simulink model "DebuggingModel_1"  (R2022b)
settings: Solver=VariableStepAuto  StartTime=0.0  StopTime=10.0  RelTol=1e-3
model workspace (MAT data in the model file):
  accumulated_data = Simulink.Signal
  accumulated_data.DataType = 'auto'
  accumulated_data.Dimensions = -1
  accumulated_data.DimensionsMode = 'auto'
  accumulated_data.Complexity = 'auto'
  accumulated_data.SampleTime = -1
  accumulated_data.SamplingMode = 'auto'
  lambda_cost = Simulink.Signal
  lambda_cost.DataType = 'double'
  lambda_cost.Dimensions = -1
  lambda_cost.DimensionsMode = 'auto'
  lambda_cost.Complexity = 'auto'
  lambda_cost.SampleTime = -1
  lambda_cost.SamplingMode = 'auto'
  lambda_cost.InitialValue = '0'
  total_cost = Simulink.Signal
  total_cost.DataType = 'auto'
  total_cost.Dimensions = -1
  total_cost.DimensionsMode = 'auto'
  total_cost.Complexity = 'auto'
  total_cost.SampleTime = -1
  total_cost.SamplingMode = 'auto'
  total_time = Simulink.Signal
  total_time.DataType = 'auto'
  total_time.Dimensions = -1
  total_time.DimensionsMode = 'auto'
  total_time.Complexity = 'auto'
  total_time.SampleTime = -1
  total_time.SamplingMode = 'auto'
libraries: VACLib x5
settings Model: Creator=KarlO  LastModifiedBy=KarlO

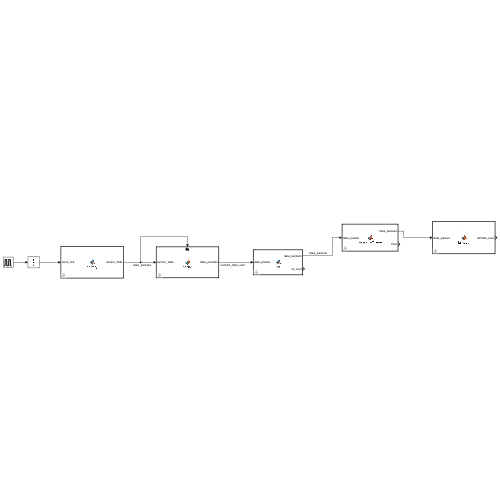
[thumbnail: Simulink's stored preview of the top-level diagram]
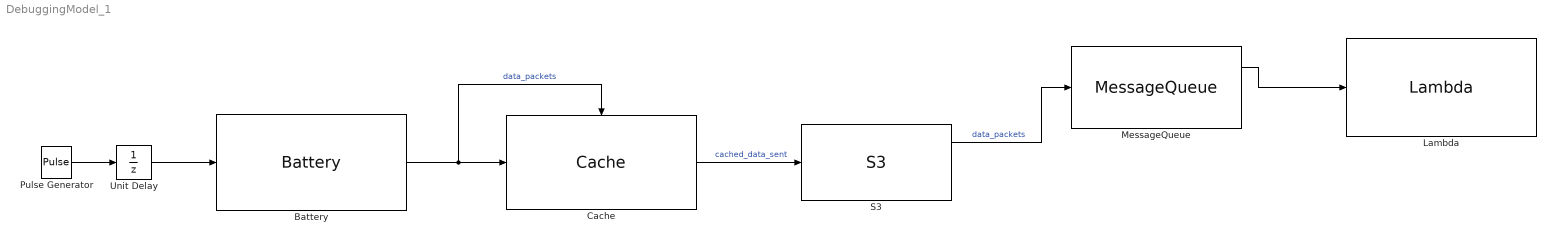
== system DebuggingModel_1 ==
  Battery : VACLib/Sources/Battery  sensor_data_size=8
      settings: LibrarySourceBlock=|
      | simulink/User-Defined
      | Functions/MATLAB Function
  Cache : VACLib/Vehicle Components/Cache  cache_size=8
      settings: LibrarySourceBlock=|
      | simulink/User-Defined
      | Functions/MATLAB Function
  Lambda : VACLib/AWS Components/Lambda  no_instances=1
      settings: LibrarySourceBlock=|
      | simulink/User-Defined
      | Functions/MATLAB Function
  MessageQueue : VACLib/AWS Components/MessageQueue  queue_size=32
      settings: LibrarySourceBlock=|
      | simulink/User-Defined
      | Functions/MATLAB Function
  Pulse Generator : DiscretePulseGenerator  PulseType=Time based  PulseWidth=50
  S3 : VACLib/AWS Components/S3  consistency=1
      settings: LibrarySourceBlock=|
      | simulink/User-Defined
      | Functions/MATLAB Function
  Unit Delay : UnitDelay  SampleTime=-1  HasFrameUpgradeWarning=on
  wires:
  Unit Delay/1 -> Battery/1
  Pulse Generator/1 -> Unit Delay/1
  Battery/1 -> Cache/1, Cache/Trigger  "data_packets"
  Cache/1 -> S3/1  "cached_data_sent"
  S3/1 -> MessageQueue/1  "data_packets"
  MessageQueue/1 -> Lambda/1
